simulink model "LQR_DUE_SIMO_SystemBlock"  (R2019a)
settings: Solver=FixedStepAuto  StartTime=0.0  StopTime=120  RelTol=1e-3  EnableMultiTasking=on
undefined symbols (not defined in the file): A, B, C, Ci, D, DiscIntNeverNeededParam, Discrete, i0, K, R, sigbuilder_block, Time, Tss, u0, y0
libraries: arduinolib x2, ctrlSharedLib x1
settings Model: SimulationMode=external  ExtModeTrigDuration=2  Creator=Jakub  LastModifiedBy=jakub
settings OptimizationCC: EnhancedBackFolding=on  PassReuseOutputArgsAs=Individual arguments  MaxStackSize=64  OptimizeBlockOrder=speed  DifferentSizesBufferReuse=on  OptimizationCustomize=off
settings DebuggingCC: ParameterTunabilityLossMsg=error
settings HardwareCC: ProdBitPerPointer=32  ProdBitPerSizeT=32  ProdBitPerPtrDiffT=32  ProdLargestAtomicInteger=Long  ProdLargestAtomicFloat=Double  ProdWordSize=32  ProdHWDeviceType=ARM Compatible->ARM Cortex
settings SFSimCC: MATLABDynamicMemAlloc=off
settings RTWCC: SystemTargetFile=ert.tlc  HardwareBoard=Arduino Due  TLCOptions=-aInlineSetEventsForThisBaseRateFcn=TLC_FALSE -aSuppressMultiTaskScheduler=TLC_FALSE -aRateBasedStepFcn=1  TemplateMakefile=ert_default_tmf  GenerateReport=on  Toolchain=Arduino ARM  BuildConfiguration=Faster Runs  IncludeHyperlinkInReport=on  LaunchReport=on  GenerateTraceInfo=on  GenerateTraceReport=on  GenerateTraceReportSl=on  GenerateTraceReportSf=on  GenerateTraceReportEml=on
settings CodeAppCC: ForceParamTrailComments=on  IgnoreCustomStorageClasses=off  OperatorAnnotations=on  SimulinkDataObjDesc=on  SFDataObjDesc=on  InsertBlockDesc=on
settings ERTTargetCC: SupportContinuousTime=on  SupportVariableSizeSignals=on  ExtModeStaticAllocSize=24576

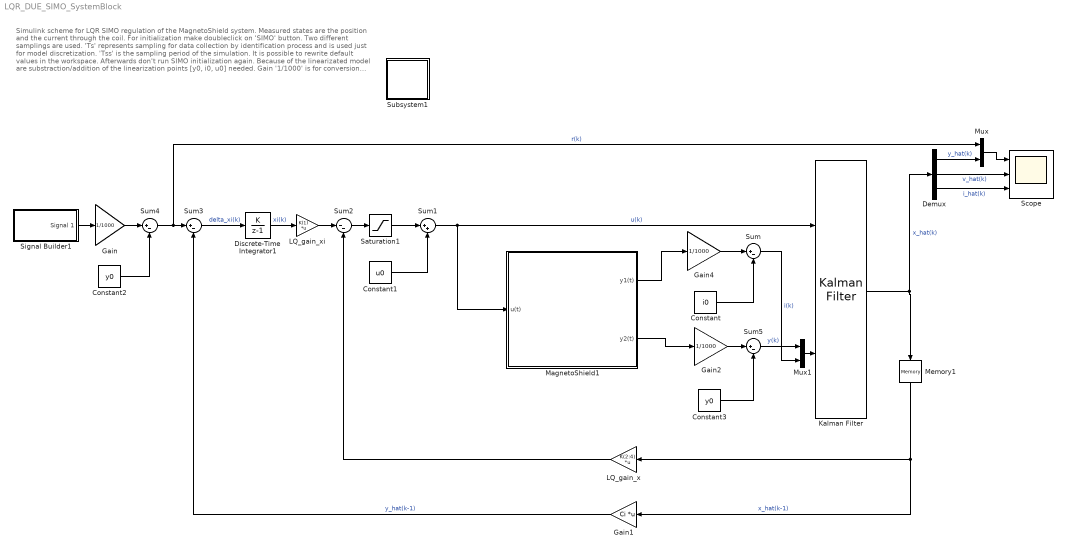
== system LQR_DUE_SIMO_SystemBlock ==
  note: Simulink scheme for LQR SIMO regulation of the MagnetoShield system. Measured states are the position
      | and the current through the coil.
      | For initialization make doubleclick on 'SIMO' button.
      |
      | Two different samplings are used. 'Ts' represents sampling for data collection by identification process
      | and is used just for model discretization. 'Tss' is the sampling period of the simulation.
      | It is possible to rewrite default values in the workspace. Afterwards don't run SIMO initialization again.
      |
      | Because of the linearizated model are substraction/addition of the linearization points [y0, i0, u0] needed.
      | Gain '1/1000' is for conversion [mm]->[m] and [mA]->[A].
      |
      | Memory block needed to avoid 'algebraic loop' error.
  Constant : Constant  Value=i0
  Constant1 : Constant  Value=u0
  Constant2 : Constant  Value=y0
  Constant3 : Constant  Value=y0
  Demux : Demux  Outputs=3
  Discrete-Time Integrator1 : DiscreteIntegrator  IntegratorMethod=Accumulation: Forward Euler  SampleTime=Tss  LimitOutput=on  UpperSaturationLimit=1  LowerSaturationLimit=-1  ICPrevOutput=DiscIntNeverNeededParam  ICPrevScaledInput=DiscIntNeverNeededParam
  Gain : Gain  Gain=1/1000
  Gain1 : Gain  Gain=Ci  Multiplication=Matrix(K*u)
  Gain2 : Gain  Gain=1/1000
  Gain4 : Gain  Gain=1/1000
  Kalman Filter : ctrlSharedLib/Kalman Filter  TimeDomain=Discrete-Time  UseCurrentEstimator=on  ModelSource=Individual A, B, C, D matrices  ModelSourceVariable=ss(0.95,1,1,0,1)  A=A  B=B  C=C  D=D  NumberOfStates=1  NumberOfInputs=1  NumberOfOutputs=1  InitialEstimateSource=Dialog  X0=0  P0=10  UseK=off  UseGH=off  NumberOfProcessNoiseInputs=1  G=1  TimeInvariantG=on  H=0  TimeInvariantH=on  Q=Q  TimeInvariantQ=on  R=R  TimeInvariantR=on  N=0  TimeInvariantN=on  AddInputPort=on  AddEnablePort=off  OutputEstimatedY=off  OutputP=off  Ts=-1
  LQ_gain_x : Gain  Gain=K(2:4)  Multiplication=Matrix(K*u)
  LQ_gain_xi : Gain  Gain=K(1)  Multiplication=Matrix(K*u)
  MagnetoShield1 : Subsystem  AncestorBlock=MagnetoLibrary/MagnetoShield  mask{Board=DUE, PositionType=Distance [mm], chackbox=on, Ts=Tss}
      mask prompts: Board "Type of the Arduino board"; PositionType "Position measured in:"; chackbox "Execute calibration at the biginning of the simulation"; Ts "Sampling period [s]"
      mask help:
      | The block represents MagnetoShield system. On the input is a control signal in the form of voltage expected (values in the range 0 - 12 V).
      | Outputs are system states - Position (y1) and Current (y2). The position is possible to measure in milimeters or in percent.
      | In the case of the closed loop control, on the feedback signals to use 'Memory' block is recomended.
      mask init:
      | mask_popup = get_param(gcb,'Board'); % which popup is choosen
      | % path to the I2C Write block
      | system = gcb;
      | way = strcat(system,'/ActuatorWrite');
      | % set Module based on Arduino type
      | if strcmp(mask_popup(1),'U')
      |     set_param(way,'Board','UNO/MEGA'); % Uno/Mega - module 0
      | elseif strcmp(mask_popup(1),'D')
      |     set_param(way,'Board','DUE'); % Due - module 1
      | end
      settings: CopyFcn=set_param(gcb, 'LinkStatus', 'inactive')
      mask TypeOptions Board: UNO/MEGA | DUE
      mask TypeOptions PositionType: Distance [mm] | Percents [%]
      mask DialogControl DescGroupVar Prompt: MagnetoShield block
      mask DialogControl ParameterGroupVar Prompt: Arduino board
      mask DialogControl Container5 Prompt: Parameters
      mask Display: image('assets\MagnetoFig\MagnetoShield.svg');
  Memory1 : Memory  InheritSampleTime=on
  Mux : Mux  Inputs=2
  Mux1 : Mux  Inputs=2
  Saturation1 : Saturate  UpperLimit=12-u0  LowerLimit=0-u0
  Scope : Scope  NumInputPorts=3
  Signal Builder1 : Subsystem  Tag=STV Subsys  LoadFcn=sigbuilder_block('load');  StartFcn=sigbuilder_block('start');  StopFcn=sigbuilder_block('stop');  ClipboardFcn=sigbuilder_block('clipboard');  mask(Sigbuilder block){tuvar=[0:10]}
      mask help: Simulink:masks:SigbuilderBlock_MD
      mask init:
      | if ~strcmp(get_param(bdroot(gcbh),'SimulationStatus'),'stopped') tuvar = sigbuilder_block('maskInit'); end
      settings: CopyFcn=sigbuilder_block('copy');  DeleteFcn=sigbuilder_block('delete');  ModelCloseFcn=sigbuilder_block('modelClose');  PreSaveFcn=sigbuilder_block('preSave');  PauseFcn=sigbuilder_block('pause');  ContinueFcn=sigbuilder_block('continue');  NameChangeFcn=sigbuilder_block('namechange');  OpenFcn=sigbuilder_block('open',[61.8 52.2 1012.8 447.6 ]);  CloseFcn=sigbuilder_block('close');
      mask Display: plot(0, 0, 100, 100,[2, 2, 32, 32, 2], [68, 8, 8, 68, 68],[32, 2], [38, 38], [32, 19, 2],[53, 60, 44], [32, 17, 17, 2],[16, 16, 31, 31]);txt = getActiveGroup(gcbh);text(2, 100, txt,'verticalAlignment', 'top');
  Subsystem1 : Subsystem
      settings: OpenFcn=|
      | load '../../../matlab/examples/MagnetoShield/MagnetoShield_Models_Greybox_SS';
      | %% MagnetoShield - LQR simulation and control initialization for Simulink
      | 
      | order = 'SIMO';                 % SISO - position / SIMO - position & current
      | Tss = 0.002;                     % Sampling
      | 
      | % Matrices extraction from model
      | modeld=c2d(model,Ts);           % Discretized linear state-space model
      | A = modeld.a;                   % Extract A
      | B = modeld.b;                   % Extract B
      | Ci = [1 0 0];                   % Position is measured for integrator 'xi' computation
      | D = 0;
      | 
      | % Discrete augmented model with integrator state - unstable, unobservable
      | Ai = [1 -Ci;
      |       zeros(3,1) A];
      | Bi = [0;B];
      | 
      | % LQ gain computation
      | Qlq=diag([70 100 20 40]);      % State penalty matrix
      | Rlq=0.1;                       % Input penalty matrix
      | K=dlqr(Ai,Bi,Qlq,Rlq);         % LQ gain for system states
      | 
      | 
      | % Measurement matrices of state-space and Kalman filter gains
      | if order == 'SISO'                  % Setup if just position is measured
      |     C = [1 0 0];
      |     D = 0;
      |     Q = diag([0.0001, 100, 100]);   % Penalty of the model for Kalman filter
      |     R = 0.001;                     % Penalty of measurement for Kalman filter
      | 
      | elseif order == 'SIMO'             % Setup if position and current are measured
      |     C = [1 0 0;0 0 1];
      |     D = [0;0];
      |     Q = diag([0.0001, 100, 80]);   % Penalty of the model for Kalman filter
      |     R = [0.001, 0.01];             % Penalty of measurement for Kalman filter
      | end
      mask Display: disp('SIMO')
  Sum{,3..5} (4 alike) : Sum  Inputs=|+-
  Sum1 : Sum  Inputs=|++
  Sum2 : Sum  Inputs=|--
  wires:
  Kalman Filter/1 -> Demux/1, Memory1/1  "x_hat(k)"
  LQ_gain_xi/1 -> Sum2/1
  Sum2/1 -> Saturation1/1
  LQ_gain_x/1 -> Sum2/2
  MagnetoShield1/1(y1(t)) -> Gain4/1
  Discrete-Time Integrator1/1 -> LQ_gain_xi/1  "xi(k)"
  Sum3/1 -> Discrete-Time Integrator1/1  "delta_xi(k)"
  Gain4/1 -> Sum/1
  Sum/1 -> Mux1/2  "i(k)"
  Constant/1 -> Sum/2
  Saturation1/1 -> Sum1/1
  Sum1/1 -> MagnetoShield1/1(u(t)), Kalman Filter/1  "u(k)"
  Constant1/1 -> Sum1/2
  Signal Builder1/1(Signal 1) -> Gain/1
  Constant2/1 -> Sum4/2
  Gain/1 -> Sum4/1
  Sum4/1 -> Mux/1, Sum3/1  "r(k)"
  Gain1/1 -> Sum3/2  "y_hat(k-1)"
  Demux/1 -> Mux/2  "y_hat(k)"
  Mux/1 -> Scope/1
  Demux/2 -> Scope/2  "v_hat(k)"
  Demux/3 -> Scope/3  "i_hat(k)"
  Mux1/1 -> Kalman Filter/2
  MagnetoShield1/2(y2(t)) -> Gain2/1
  Gain2/1 -> Sum5/1
  Constant3/1 -> Sum5/2
  Sum5/1 -> Mux1/1  "y(k)"
  Memory1/1 -> LQ_gain_x/1, Gain1/1  "x_hat(k-1)"

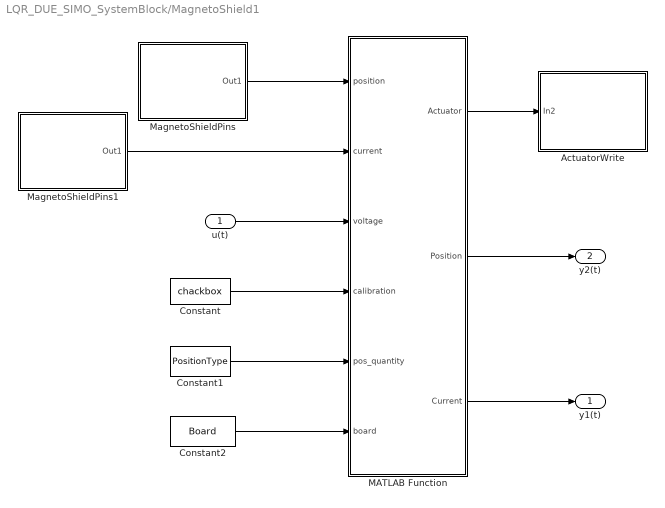
== system LQR_DUE_SIMO_SystemBlock/MagnetoShield1 ==
  u(t) : Inport
  ActuatorWrite : Subsystem  AncestorBlock=MagnetoLibrary/ActuatorWrite  mask{Board=DUE, Units=Volts}
      mask prompts: Board "Type of the Arduino board"; Units "Input unite"
      mask help:
      | ActuatorWrite block allows to set desired voltage value on the electromagnet. The desired value can be expresed as voltage, percentage of maximal possible voltage or as a value of the magnetic field in Gausses as well.
      | This block converts input control signal into suficient form (16-bit number) and writes the information on the MCP4725-DAC converter.
      | Maximal voltage range: 0-12 V
      mask init:
      | mask_popup = get_param(gcb,'Board'); % which popup is choosen
      | % path to the I2C Write block
      | system = gcb;
      | way = strcat(system,'/I2C Write UNO');
      | % set Module based on Arduino type
      | if strcmp(mask_popup(1),'U')
      |     set_param(way,'I2CModule','0'); % Uno/Mega - module 0
      | elseif strcmp(mask_popup(1),'D')
      |     set_param(way,'I2CModule','1'); % Due - module 1
      | end
      settings: CopyFcn=set_param(gcb, 'LinkStatus', 'inactive')
      mask TypeOptions Board: UNO/MEGA | DUE
      mask TypeOptions Units: Volts | Percents | DAC levels
      mask DialogControl DescGroupVar Prompt: ActuatorWrite block
      mask Display: image('assets\MagnetoFig\ActuatorWrite.svg');
  Constant : Constant  Value=chackbox  SampleTime=Ts
  Constant1 : Constant  Value=PositionType  SampleTime=Ts
  Constant2 : Constant  Value=Board  SampleTime=Ts
  MATLAB Function : MATLAB Function  TreatAsAtomicUnit=on
  MagnetoShieldPins : Subsystem  AncestorBlock=MagnetoLibrary/MagnetoShieldPins  mask{PIN=Hall sensor pin (A3), sampling=Ts}
      mask prompts: PIN "Choose pin"; sampling "Sampling period [s]"
      mask help:
      | User can choose a pin on which the data should be processed.
      | >Hall sensor pin - data about the possition of the levitating magnet.
      | >Voltage pin - voltage on the electromagnet
      | >Current pin - current crossing the electromagnet
      | >Reference pin - data from potentiometer, used as adjustable analog reference
      | (output = double)
      mask init:
      | letter = PIN;
      | if letter==1
      | path='assets\MagnetoFig\Pins\hpin.svg';
      | elseif letter==2
      | path='assets\MagnetoFig\Pins\vpin.svg';
      | elseif letter==3
      | path='assets\MagnetoFig\Pins\cpin.svg';
      | else
      | path='assets\MagnetoFig\Pins\ppin.svg';    
      | end
      settings: CopyFcn=set_param(gcb, 'LinkStatus', 'inactive')
      mask TypeOptions PIN: Hall sensor pin (A3) | Voltage pin (A1) | Current pin (A2) | Reference pin (A0)
      mask Callback PIN:
      | mask_popup = get_param(gcb,'PIN'); % which popup is choosen
      | % path to the I2C Write block
      | system = gcb;
      | way = strcat(system,'/Analog Input');
      | % set Module based on Arduino type
      | if strcmp(mask_popup(1),'H')
      |     set_param(way,'pinNumber','3'); % Uno/Mega - module 0
      | elseif strcmp(mask_popup(1),'V')
      |     set_param(way,'pinNumber','1'); % Due - module 1
      | elseif strcmp(mask_popup(1),'C')
      |     set_param(way,'pinNumber','2'); % Due - module 1
      | elseif strcmp(mask_popup(1),'R')
      |     set_param(way,'pinNumber','0'); % Due - module 11
      | end
      mask DialogControl DescGroupVar Prompt: MagnetoShieldPins block
      mask Display: image(path);
  MagnetoShieldPins1 : Subsystem  AncestorBlock=MagnetoLibrary/MagnetoShieldPins  mask{PIN=Current pin (A2), sampling=Ts}
      mask prompts: PIN "Choose pin"; sampling "Sampling period [s]"
      mask help:
      | User can choose a pin on which the data should be processed.
      | >Hall sensor pin - data about the possition of the levitating magnet.
      | >Voltage pin - voltage on the electromagnet
      | >Current pin - current crossing the electromagnet
      | >Reference pin - data from potentiometer, used as adjustable analog reference
      | (output = double)
      mask init: same as LQR_DUE_SIMO_SystemBlock/MagnetoShield1/MagnetoShieldPins
      settings: CopyFcn=set_param(gcb, 'LinkStatus', 'inactive')
      mask TypeOptions PIN: Hall sensor pin (A3) | Voltage pin (A1) | Current pin (A2) | Reference pin (A0)
      mask Callback PIN:
      | mask_popup = get_param(gcb,'PIN'); % which popup is choosen
      | % path to the I2C Write block
      | system = gcb;
      | way = strcat(system,'/Analog Input');
      | % set Module based on Arduino type
      | if strcmp(mask_popup(1),'H')
      |     set_param(way,'pinNumber','3'); % Uno/Mega - module 0
      | elseif strcmp(mask_popup(1),'V')
      |     set_param(way,'pinNumber','1'); % Due - module 1
      | elseif strcmp(mask_popup(1),'C')
      |     set_param(way,'pinNumber','2'); % Due - module 1
      | elseif strcmp(mask_popup(1),'R')
      |     set_param(way,'pinNumber','0'); % Due - module 11
      | end
      mask DialogControl DescGroupVar Prompt: MagnetoShieldPins block
      mask Display: image(path);
  y1(t) : Outport  VectorParamsAs1DForOutWhenUnconnected=off
  y2(t) : Outport  Port=2  VectorParamsAs1DForOutWhenUnconnected=off
  wires:
  MATLAB Function/3(Current) -> y1(t)/1
  Constant2/1 -> MATLAB Function/6(board)
  Constant1/1 -> MATLAB Function/5(pos_quantity)
  Constant/1 -> MATLAB Function/4(calibration)
  MagnetoShieldPins1/1(Out1) -> MATLAB Function/2(current)
  u(t)/1 -> MATLAB Function/3(voltage)
  MATLAB Function/2(Position) -> y2(t)/1
  MagnetoShieldPins/1(Out1) -> MATLAB Function/1(position)
  MATLAB Function/1(Actuator) -> ActuatorWrite/1(In2)

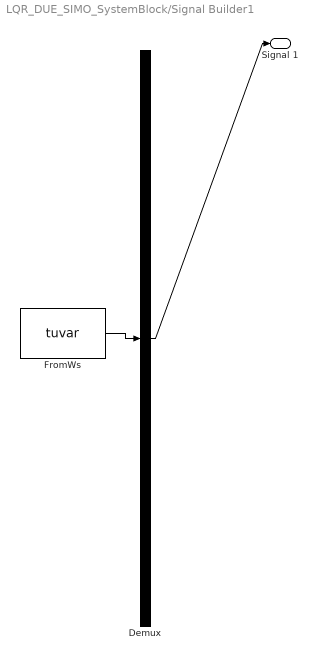
== system LQR_DUE_SIMO_SystemBlock/Signal Builder1 ==
  Demux : Demux  Tag=STV Demux  Outputs=1
      settings: DisplayOption=none
  FromWs : FromWorkspace  Tag=STV FromWs  VariableName=tuvar
      SigBuilderData=|
      | common.afterFinalStr = 'Extrapolate'
      | common.sampleTime = 0
      | dataSet.timeRange = [0 120]
      | dataSet.name = 'Group 1'
      | sbobj.Groups.Name = 'Group 1'
      | sbobj.Groups.Signals.Name = 'Signal 1'
      | sbobj.Groups.Signals.XData = [0 5 5 10 15 15 20 25 25 30 35 35 40 45 45 50 55 55 60 65 70 70 75 80 85 85 90 95 100 105 110 115 115 120]
      | sbobj.Groups.Signals.YData = [17 17 16.5 16.5 16.5 15.5 15.5 15.5 14.5 14.5 14.5 13.5 13.5 13.5 12.5 12.5 12.5 16 16 16 16 13.5 13.5 13.5 13.5 15 15 15 17 12 14.5 14.5 17 17]
      | sbobj.Groups.TimeRange = [0 120]
  Signal 1 : Outport  Tag=STV Outport  VectorParamsAs1DForOutWhenUnconnected=off
  wires:
  FromWs/1 -> Demux/1
  Demux/1 -> Signal 1/1

== system LQR_DUE_SIMO_SystemBlock/Subsystem1 ==

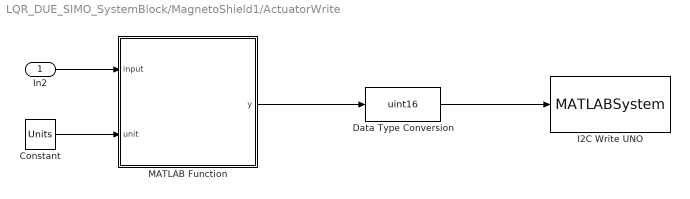
== system LQR_DUE_SIMO_SystemBlock/MagnetoShield1/ActuatorWrite ==
  In2 : Inport
  Constant : Constant  Value=Units
  Data Type Conversion : DataTypeConversion  OutDataTypeStr=uint16
  I2C Write UNO : MATLABSystem  AncestorBlock=arduinolib/I2C Write  InitFcn=|  System=codertarget.arduinobase.internal.arduinoI2CWrite  I2CModule=1  Mode=Master  SlaveAddress=96  SlaveByteOrder=BigEndian  Direction=Transmitter  RegisterAddressMode=off  RegisterAddress=0  SlaveDataType=uint8  DataLength=1  NoAck=off  RepeatedStart=off  OutputStatus=off  blockPlatform=ARDUINO
      | codertarget.arduinobase.blocks.registerI2CBlock(gcbh);
      | codertarget.arduinobase.blocks.arduinoBlockInitFcnCallback(gcbh);
      mask Type: I2C Write
      mask Display:
      | color('white');
      | plot([100,100,100,100],[100,100,100,100]);
      | plot([0,0,0,0],[0,0,0,0]);
      | color('blue');
      | text(99, 92, 'ARDUINO', 'horizontalAlignment', 'right');
      | color('black');
      | text(50,60,'\fontsize{12}\bfI2C','texmode','on','horizontalAlignment','center','verticalAlignment','middle');
      | text(50,40,'\fontsize{10}\bfMaster Write','texmode','on','horizontalAlignment','center','verticalAlignment','middle');
      | text(50,15,'Slave: 0x60' ,'horizontalAlignment', 'center');
      | port_label('input',1,'Data');
  MATLAB Function : MATLAB Function  TreatAsAtomicUnit=on
  wires:
  In2/1 -> MATLAB Function/1(input)
  Constant/1 -> MATLAB Function/2(unit)
  Data Type Conversion/1 -> I2C Write UNO/1
  MATLAB Function/1(y) -> Data Type Conversion/1

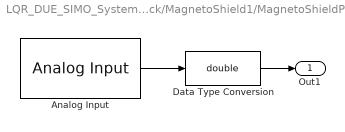
== system LQR_DUE_SIMO_SystemBlock/MagnetoShield1/MagnetoShieldPins ==
  Analog Input : arduinolib/Analog Input  pinNumber=3  ReadResultsOnly=off  ConversionTriggerSource=Software  ExternalTriggerType=uint32(0)  OutputDataType=uint16  EnableConversionCompleteNotify=off  EnableOuputStatus=off  SampleTime=sampling  blockPlatform=arduino
  Data Type Conversion : DataTypeConversion  OutDataTypeStr=double
  Out1 : Outport  VectorParamsAs1DForOutWhenUnconnected=off
  wires:
  Analog Input/1 -> Data Type Conversion/1
  Data Type Conversion/1 -> Out1/1

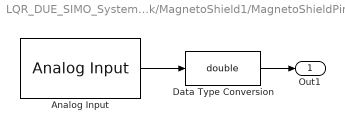
== system LQR_DUE_SIMO_SystemBlock/MagnetoShield1/MagnetoShieldPins1 ==
  Analog Input : arduinolib/Analog Input  pinNumber=2  ReadResultsOnly=off  ConversionTriggerSource=Software  ExternalTriggerType=uint32(0)  OutputDataType=uint16  EnableConversionCompleteNotify=off  EnableOuputStatus=off  SampleTime=sampling  blockPlatform=arduino
  Data Type Conversion : DataTypeConversion  OutDataTypeStr=double
  Out1 : Outport  VectorParamsAs1DForOutWhenUnconnected=off
  wires:
  Analog Input/1 -> Data Type Conversion/1
  Data Type Conversion/1 -> Out1/1

== matlab function LQR_DUE_SIMO_SystemBlock/MagnetoShield1/ActuatorWrite/MATLAB Function ==
  data: input input; y output; unit input
function y = fcn(input,unit)

if unit==1 % voltage
    y = 4095/12*input;
elseif unit==2 % percents
    y = 4095/100*input;
elseif unit==3 % dac levels
    y = input;
else
     y = 0; % needed instance
end
% secures that 12-bit number will not overcross a size boundary
if y>4095
    y=4095;
elseif y<0
    y=0;
end

end

== matlab function LQR_DUE_SIMO_SystemBlock/MagnetoShield1/MATLAB Function ==
  data: position input; Actuator output; current input; Position output; voltage input; calibration input; Current output; pos_quantity input; board input
function [Actuator,Position,Current] = fcn(position,current,voltage,calibration,pos_quantity,board)
persistent adcMAX adcMIN p_d1 p_d2 counter calib ARES3V3 A1302_SENSITIVITY;
if isempty(counter)
         p_d1 = 3.233100;
         p_d2 = 0.220571;
         counter = 0;
         calib = calibration;
         if calibration==1
            adcMAX = 300;
            adcMIN = 300;
         else
            adcMAX = 2526;
            adcMIN = 112;
         end
         A1302_SENSITIVITY = 769.23;
         if board==1                 % choose board
            ARES3V3 = 3.3/1023;     % UNO
         else 
            ARES3V3 = 3.3/4095;     % DUE
         end
end
% CALIBRATION PHASE
if calib == 1
    % Minimal ADC level measured on the hall sensor
    if counter<=500
        Actuator = 0;
        if position<adcMIN
            adcMIN = position;
        end
    % Maximal ADC level measured on the hall sensor    
    elseif counter>500 && counter<=1000
        Actuator = 12;
        if position>adcMAX
            adcMAX = position; 
        end
    % Calibration calculations
    else
        Actuator = 0;
        p_d2 = log(17/12)/log((2.5-adcMIN*ARES3V3)*A1302_SENSITIVITY/((2.5-adcMAX*ARES3V3)*A1302_SENSITIVITY));
        p_d1 = 12/((2.5-adcMAX*ARES3V3)*A1302_SENSITIVITY)^p_d2;
        % Time 500 samples to settle down the magnet
        if counter>1500
            calib = 0;
        end
    end
    Position = 0;   % default outputs during calibration
    Current = 0;
    counter = counter+1;
% CONTROL PHASE
elseif calib == 0
    Actuator = voltage;
    % position measured in:
    if pos_quantity==2  % percents
        Position = (position-adcMIN)*100/(adcMAX-adcMIN);
    else            % distance
        gauss = (2.5-position*ARES3V3)*A1302_SENSITIVITY;
        Position = p_d1*gauss^p_d2;
    end
    % current measurement
    Current = current*ARES3V3*33.333333; %Igain = 33.333333
% ERROR SIGNALIZATION    
else
    Actuator = 42;
    Position = 42;
    Current = 42;
end
